simulink model "Test_Byte_Multiplexer_16_to_1_DirSel"  (Simulink 8.7)
settings: Solver=ode45  StartTime=0.0  StopTime=len  RelTol=1e-3
libraries: Miscellaneous x17, commutil2 x1, Byte_Multiplexers_Lib x1
settings Model: Creator=N  LastModifiedBy=Jozko Mrkvicka
settings DataIOCC: LimitDataPoints=off
settings DebuggingCC: UnderspecifiedInitializationDetection=Simplified  MergeDetectMultiDrivingBlocksExec=error
settings HardwareCC: ProdBitPerPointer=64  ProdLargestAtomicFloat=Float  ProdIntDivRoundTo=Zero  ProdEndianess=LittleEndian  ProdHWDeviceType=Intel->x86-64 (Windows64)
settings ModelReferenceCC: PropagateSignalLabelsOutOfModel=on

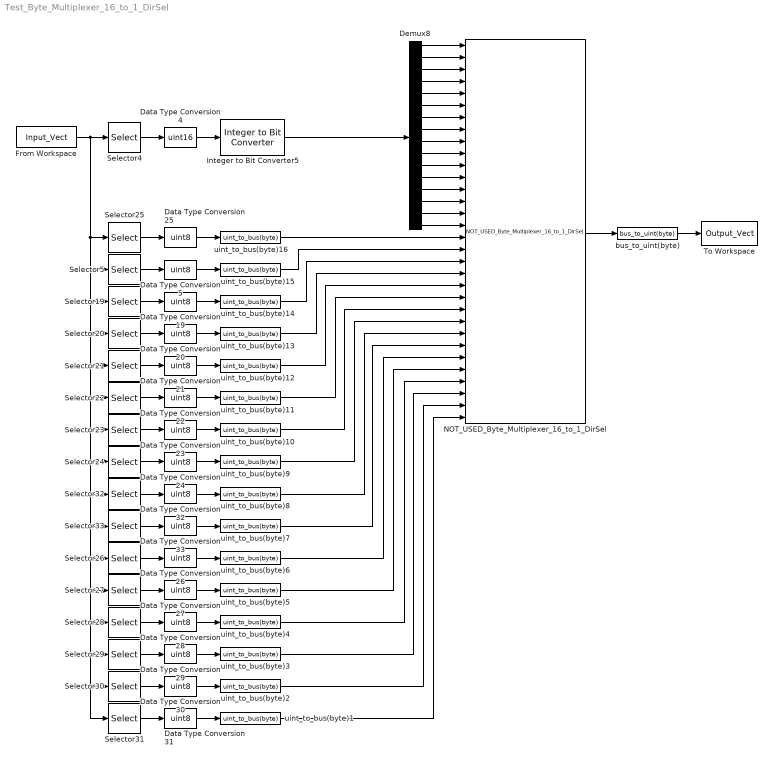
== system Test_Byte_Multiplexer_16_to_1_DirSel ==
  Data Type Conversion{5,19..33} (16 alike) : DataTypeConversion  OutDataTypeStr=uint8
  Data Type Conversion4 : DataTypeConversion  OutDataTypeStr=uint16
  Demux8 : Demux  Outputs=16
  From Workspace : FromWorkspace  VariableName=Input_Vect  SampleTime=1  Interpolate=off  OutputAfterFinalValue=Holding final value
  Integer to Bit Converter5 : commutil2/Integer to Bit Converter  nbits=16  signedInputValues=Unsigned  bitOrder=MSB first  outDtype=boolean
  NOT_USED_Byte_Multiplexer_16_to_1_DirSel : Byte_Multiplexers_Lib/Byte_Multiplexers_Lib/NOT_USED_Byte_Multiplexer_16_to_1_DirSel
  Selector19 : Selector  IndexMode=Zero-based  InputPortWidth=17  IndexOptions=Index vector (dialog)  Indices=3  OutputSizes=1
  Selector20 : Selector  IndexMode=Zero-based  InputPortWidth=17  IndexOptions=Index vector (dialog)  Indices=4  OutputSizes=1
  Selector21 : Selector  IndexMode=Zero-based  InputPortWidth=17  IndexOptions=Index vector (dialog)  Indices=5  OutputSizes=1
  Selector22 : Selector  IndexMode=Zero-based  InputPortWidth=17  IndexOptions=Index vector (dialog)  Indices=6  OutputSizes=1
  Selector23 : Selector  IndexMode=Zero-based  InputPortWidth=17  IndexOptions=Index vector (dialog)  Indices=7  OutputSizes=1
  Selector24 : Selector  IndexMode=Zero-based  InputPortWidth=17  IndexOptions=Index vector (dialog)  Indices=8  OutputSizes=1
  Selector25 : Selector  IndexMode=Zero-based  InputPortWidth=17  IndexOptions=Index vector (dialog)  Indices=1  OutputSizes=1
  Selector26 : Selector  IndexMode=Zero-based  InputPortWidth=17  IndexOptions=Index vector (dialog)  Indices=11  OutputSizes=1
  Selector27 : Selector  IndexMode=Zero-based  InputPortWidth=17  IndexOptions=Index vector (dialog)  Indices=12  OutputSizes=1
  Selector28 : Selector  IndexMode=Zero-based  InputPortWidth=17  IndexOptions=Index vector (dialog)  Indices=13  OutputSizes=1
  Selector29 : Selector  IndexMode=Zero-based  InputPortWidth=17  IndexOptions=Index vector (dialog)  Indices=14  OutputSizes=1
  Selector30 : Selector  IndexMode=Zero-based  InputPortWidth=17  IndexOptions=Index vector (dialog)  Indices=15  OutputSizes=1
  Selector31 : Selector  IndexMode=Zero-based  InputPortWidth=17  IndexOptions=Index vector (dialog)  Indices=16  OutputSizes=1
  Selector32 : Selector  IndexMode=Zero-based  InputPortWidth=17  IndexOptions=Index vector (dialog)  Indices=9  OutputSizes=1
  Selector33 : Selector  IndexMode=Zero-based  InputPortWidth=17  IndexOptions=Index vector (dialog)  Indices=10  OutputSizes=1
  Selector4 : Selector  IndexMode=Zero-based  InputPortWidth=17  SampleTime=1  IndexOptions=Index vector (dialog)  Indices=0  OutputSizes=1
  Selector5 : Selector  IndexMode=Zero-based  InputPortWidth=17  IndexOptions=Index vector (dialog)  Indices=2  OutputSizes=1
  To Workspace : ToWorkspace  VariableName=Output_Vect  SampleTime=1
  bus_to_uint(byte) : Miscellaneous/bus_to_uint(byte)
  uint_to_bus(byte){1..16} (16 alike) : Miscellaneous/uint_to_bus(byte)
  wires:
  Integer to Bit Converter5/1 -> Demux8/1
  NOT_USED_Byte_Multiplexer_16_to_1_DirSel/1 -> bus_to_uint(byte)/1
  Data Type Conversion4/1 -> Integer to Bit Converter5/1
  uint_to_bus(byte)16/1 -> NOT_USED_Byte_Multiplexer_16_to_1_DirSel/17
  uint_to_bus(byte)15/1 -> NOT_USED_Byte_Multiplexer_16_to_1_DirSel/18
  uint_to_bus(byte)14/1 -> NOT_USED_Byte_Multiplexer_16_to_1_DirSel/19
  uint_to_bus(byte)13/1 -> NOT_USED_Byte_Multiplexer_16_to_1_DirSel/20
  uint_to_bus(byte)12/1 -> NOT_USED_Byte_Multiplexer_16_to_1_DirSel/21
  uint_to_bus(byte)11/1 -> NOT_USED_Byte_Multiplexer_16_to_1_DirSel/22
  uint_to_bus(byte)10/1 -> NOT_USED_Byte_Multiplexer_16_to_1_DirSel/23
  uint_to_bus(byte)9/1 -> NOT_USED_Byte_Multiplexer_16_to_1_DirSel/24
  uint_to_bus(byte)8/1 -> NOT_USED_Byte_Multiplexer_16_to_1_DirSel/25
  uint_to_bus(byte)7/1 -> NOT_USED_Byte_Multiplexer_16_to_1_DirSel/26
  uint_to_bus(byte)6/1 -> NOT_USED_Byte_Multiplexer_16_to_1_DirSel/27
  uint_to_bus(byte)5/1 -> NOT_USED_Byte_Multiplexer_16_to_1_DirSel/28
  uint_to_bus(byte)4/1 -> NOT_USED_Byte_Multiplexer_16_to_1_DirSel/29
  uint_to_bus(byte)3/1 -> NOT_USED_Byte_Multiplexer_16_to_1_DirSel/30
  uint_to_bus(byte)2/1 -> NOT_USED_Byte_Multiplexer_16_to_1_DirSel/31
  uint_to_bus(byte)1/1 -> NOT_USED_Byte_Multiplexer_16_to_1_DirSel/32
  bus_to_uint(byte)/1 -> To Workspace/1
  Demux8/1 -> NOT_USED_Byte_Multiplexer_16_to_1_DirSel/1
  Demux8/2 -> NOT_USED_Byte_Multiplexer_16_to_1_DirSel/2
  Demux8/3 -> NOT_USED_Byte_Multiplexer_16_to_1_DirSel/3
  Demux8/4 -> NOT_USED_Byte_Multiplexer_16_to_1_DirSel/4
  Demux8/5 -> NOT_USED_Byte_Multiplexer_16_to_1_DirSel/5
  Demux8/6 -> NOT_USED_Byte_Multiplexer_16_to_1_DirSel/6
  Demux8/7 -> NOT_USED_Byte_Multiplexer_16_to_1_DirSel/7
  Demux8/8 -> NOT_USED_Byte_Multiplexer_16_to_1_DirSel/8
  Demux8/9 -> NOT_USED_Byte_Multiplexer_16_to_1_DirSel/9
  Demux8/10 -> NOT_USED_Byte_Multiplexer_16_to_1_DirSel/10
  Demux8/11 -> NOT_USED_Byte_Multiplexer_16_to_1_DirSel/11
  Demux8/12 -> NOT_USED_Byte_Multiplexer_16_to_1_DirSel/12
  Demux8/13 -> NOT_USED_Byte_Multiplexer_16_to_1_DirSel/13
  Demux8/14 -> NOT_USED_Byte_Multiplexer_16_to_1_DirSel/14
  Demux8/15 -> NOT_USED_Byte_Multiplexer_16_to_1_DirSel/15
  Demux8/16 -> NOT_USED_Byte_Multiplexer_16_to_1_DirSel/16
  Selector4/1 -> Data Type Conversion4/1
  From Workspace/1 -> Selector5/1, Selector19/1, Selector20/1, Selector21/1, Selector22/1, Selector23/1, Selector32/1, Selector33/1, Selector26/1, Selector27/1, Selector28/1, Selector29/1, Selector30/1, Selector31/1, Selector24/1, Selector25/1, Selector4/1
  Selector25/1 -> Data Type Conversion25/1
  Selector5/1 -> Data Type Conversion5/1
  Selector19/1 -> Data Type Conversion19/1
  Selector20/1 -> Data Type Conversion20/1
  Selector21/1 -> Data Type Conversion21/1
  Selector22/1 -> Data Type Conversion22/1
  Selector23/1 -> Data Type Conversion23/1
  Selector24/1 -> Data Type Conversion24/1
  Selector32/1 -> Data Type Conversion32/1
  Selector33/1 -> Data Type Conversion33/1
  Selector26/1 -> Data Type Conversion26/1
  Selector27/1 -> Data Type Conversion27/1
  Selector28/1 -> Data Type Conversion28/1
  Selector29/1 -> Data Type Conversion29/1
  Selector30/1 -> Data Type Conversion30/1
  Selector31/1 -> Data Type Conversion31/1
  Data Type Conversion31/1 -> uint_to_bus(byte)1/1
  Data Type Conversion29/1 -> uint_to_bus(byte)3/1
  Data Type Conversion30/1 -> uint_to_bus(byte)2/1
  Data Type Conversion28/1 -> uint_to_bus(byte)4/1
  Data Type Conversion27/1 -> uint_to_bus(byte)5/1
  Data Type Conversion26/1 -> uint_to_bus(byte)6/1
  Data Type Conversion33/1 -> uint_to_bus(byte)7/1
  Data Type Conversion32/1 -> uint_to_bus(byte)8/1
  Data Type Conversion24/1 -> uint_to_bus(byte)9/1
  Data Type Conversion23/1 -> uint_to_bus(byte)10/1
  Data Type Conversion22/1 -> uint_to_bus(byte)11/1
  Data Type Conversion21/1 -> uint_to_bus(byte)12/1
  Data Type Conversion20/1 -> uint_to_bus(byte)13/1
  Data Type Conversion19/1 -> uint_to_bus(byte)14/1
  Data Type Conversion5/1 -> uint_to_bus(byte)15/1
  Data Type Conversion25/1 -> uint_to_bus(byte)16/1
